simulink model "PMSG_Grid"  (R2023a)
settings: Solver=VariableStepAuto  StartTime=0.0  StopTime=4  FixedStep=1e-6  RelTol=1e-3  AbsTol=1e-3
libraries: slpidlib x6, spsabctodq0Lib x3, spsSVPWMGenerator2LevelLib x2, spsdq0toAlphaBetaZeroLib x2, spsUniversalBridgeLib x2, spsPermanentMagnetSynchronousMachineLib x1, spsPower3phInstantaneousLib x1, spspowerguiLib x1, spsSeriesRLCBranchLib x1, spsThreePhaseVIMeasurementLib x1, spsThreePhaseSourceLib x1, spsVoltageMeasurementLib x1
settings Model: Creator=MY  LastModifiedBy=MY

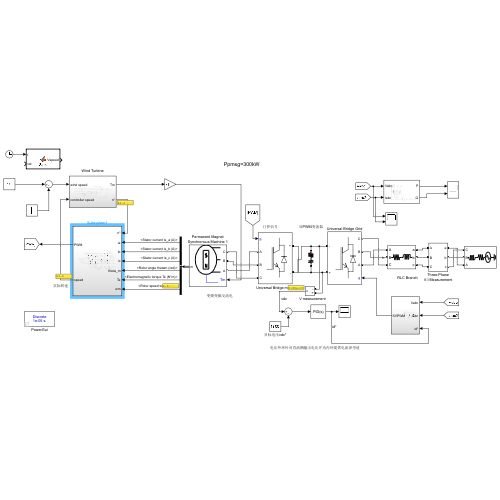
[thumbnail: Simulink's stored preview of the top-level diagram]
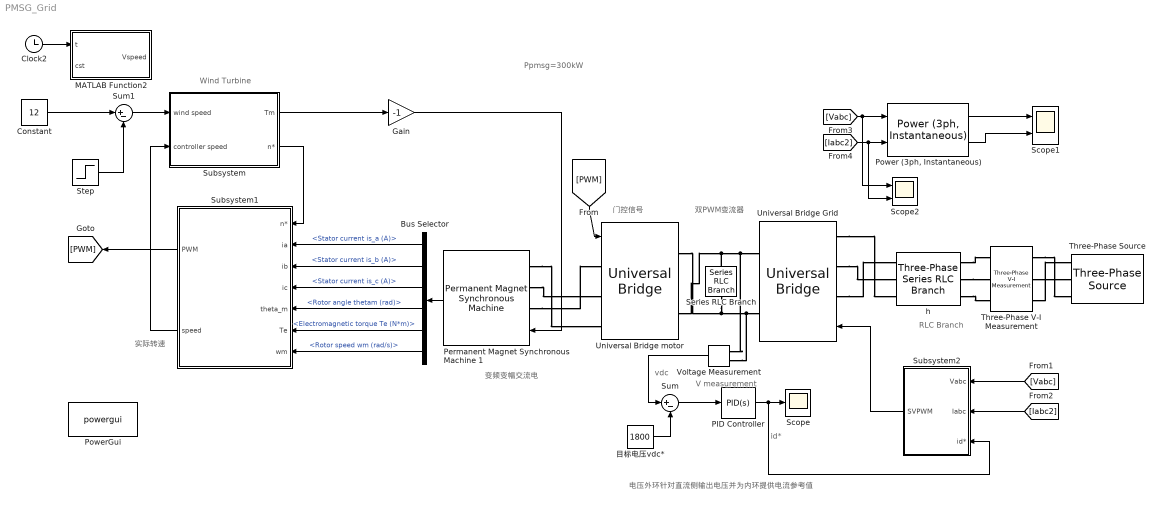
== system PMSG_Grid ==
  note: vdc
  note: 电压外环针对直流侧输出电压并为内环提供电流参考值
  note: 双PWM变流器
  note: 门控信号
  note: 变频变幅交流电
  note: 实际转速
  note: RLC Branch
  note: Ppmsg=300kW
  note: V measurement
  note: id*
  note: Wind Turbine
  Bus Selector : BusSelector  OutputSignals=Stator current is_a (A),Stator current is_b (A),Stator current is_c (A),Rotor angle thetam (rad),Electromagnetic torque Te (N*m),Rotor speed wm (rad/s)
  Clock2 : Clock
  Constant : Constant  Value=12
  Gain : Gain  Gain=-1
  MATLAB Function2 : MATLAB Function  InitFcn=""  StopFcn=""  TreatAsAtomicUnit=on
  PID Controller : slpidlib/PID Controller  Controller=PID  Form=Parallel  TimeDomain=Continuous-time  UseExternalTs=off  SampleTime=-1  IntegratorMethod=Forward Euler  FilterMethod=Forward Euler  ControllerParametersSource=internal  P=1  I=15  UseKiTs=off  D=0  N=100  UseFilter=on  TunerSelectOption=Transfer Function Based (PID Tuner App)  InitialConditionSource=internal  InitialConditionForIntegrator=0  InitialConditionForFilter=0  DifferentiatorICPrevScaledInput=0  ExternalReset=none  TrackingMode=off  Kt=1  LimitOutput=off  SatLimitsSource=internal  UpperSaturationLimit=inf  LowerSaturationLimit=-inf  LinearizeAsGain=on  AntiWindupMode=none  Kb=1  LimitIntegrator=off  UpperIntegratorSaturationLimit=inf  LowerIntegratorSaturationLimit=-inf  POutMin=[]  POutMax=[]  IOutMin=[]  IOutMax=[]  DOutMin=[]  DOutMax=[]  NOutMin=[]  NOutMax=[]  SumOutMin=[]  SumOutMax=[]  SaturationOutMin=[]  SaturationOutMax=[]  PParamMin=[]  PParamMax=[]  IParamMin=[]  IParamMax=[]  DParamMin=[]  DParamMax=[]  NParamMin=[]  NParamMax=[]  KbParamMin=[]  KbParamMax=[]  KtParamMin=[]  KtParamMax=[]  KbOutMin=[]  KbOutMax=[]  KtOutMin=[]  KtOutMax=[]  IntegratorOutMin=[]  IntegratorOutMax=[]  FilterOutMin=[]  FilterOutMax=[]  SumI1OutMin=[]  SumI1OutMax=[]  SumI2OutMin=[]  SumI2OutMax=[]  SumI3OutMin=[]  SumI3OutMax=[]  SumI4OutMin=[]  SumI4OutMax=[]  SumDOutMin=[]  SumDOutMax=[]  DifferentiatorOutMin=[]  DifferentiatorOutMax=[]  FilterDiffOutCoefMin=[]  FilterDiffOutCoefMax=[]  ReciprocalOutMin=[]  ReciprocalOutMax=[]  SumDenOutMin=[]  SumDenOutMax=[]  SumNumOutMin=[]  SumNumOutMax=[]  DivideOutMin=[]  DivideOutMax=[]  UdiffTsProdOutMin=[]  UdiffTsProdOutMax=[]  NTsProdOutMin=[]  NTsProdOutMax=[]  UintegralTsProdOutMin=[]  UintegralTsProdOutMax=[]  UngainTsProdOutMin=[]  UngainTsProdOutMax=[]  ClampingZeroOutDataTypeStr=Inherit: Inherit via back propagation  ClampingZeroOutMin=[]  ClampingZeroOutMax=[]  FilterDenConstantOutDataTypeStr=Inherit: Inherit via back propagation  FilterDenConstantOutMin=[]  FilterDenConstantOutMax=[]  PCopyOutDataTypeStr=Inherit: Inherit via back propagation  PCopyOutMin=[]  PCopyOutMax=[]  NCopyOutDataTypeStr=Inherit: Inherit via back propagation  NCopyOutMin=[]  NCopyOutMax=[]  IntegratorContinuousStateAttributes=''  IntegratorStateMustResolveToSignalObject=off  IntegratorRTWStateStorageClass=Auto  FilterContinuousStateAttributes=''  FilterStateMustResolveToSignalObject=off  FilterRTWStateStorageClass=Auto  ParallelPVariant=InternalParameters  IdealPVariant=Disabled  IVariant=InternalParameters  DVariant=InternalParameters  IntegratorVariant=Continuous  SatVariant=Disabled  AWVariant=Passthrough  PCopyVariant=Disabled  TRVariant=Disabled  FdbkBlocksVariant=Forward  IdealPFdbkVariant=Disabled  SatFdbkVariant=Disabled  DerivativeFilterVariant=ContFilter  NVariant=InternalParameters  NCopyVariant=Disabled  FilterICVariant=InternalICsFilter  IntegratorICVariant=InternalICs  ExternalResetVariant=Disabled  TRSumVariant=Passthrough  SumFdbkVariant=Disabled  SumVariant=Sum_PID  TsampFilterVariant=InternalTs  TsampNgainVariant=Passthrough  TsampIntegralVariant=Disabled_SignalSpec  ExternalSaturationOutDataTypeStr=Inherit: Same as second input
  Permanent Magnet Synchronous Machine 1 : spsPermanentMagnetSynchronousMachineLib/Permanent Magnet Synchronous Machine  NbPhases=3  FluxDistribution=Sinusoidal  RotorType=Round  MechanicalLoad=Torque Tm  PresetModel=No  ShowDetailedParameters=on  MeasurementBus=off  Resistance=0.025  Inductance=8.5e-3  dqInductances=[8.5e-3,8.5e-3]  La=0.0036  MachineConstant=Flux linkage established by magnets (V.s)  Flux=3.88889  VoltageCst=8464.3995  TorqueCst=70  Flat=120  Mechanical=[60 0.078 12 0]  PolePairs=4  InitialConditions=[0,0, 0,0]  InitialConditions5ph=[0 0 0 0 0 0]  RefAngle=90 degrees behind phase A axis (modified Park)  IterativeDiscreteModel=Trapezoidal non iterative  TsBlock=-1  TsPowergui=0
  "Power (3ph, Instantaneous)" : spsPower3phInstantaneousLib/Power (3ph, Instantaneous)
  PowerGui : spspowerguiLib/powergui  Priority=1  SimulationMode=Discrete  SampleTime=1e-5  frequency=60  Iterations=50  frequencyindice=60  Pbase=100e6  ErrMax=1e-4  UnitsV=kV  UnitsW=MW  buscounter=0  FunctionMessages=off  echomessages=off  EnableUseOfTLC=off  CurrentSourceSwitches=off  DisableSnubberDevices=off  DisableRonSwitches=off  DisableVfSwitches=off  DisplayEquations=off  AutomaticDiscreteSolvers=off  SolverType=Tustin/Backward Euler (TBE)  Interpol=off  ExternalGateDelay=off  methode=off  Ts=100  x0status=blocks  SPID=on  SwTol=0  HookPort=off  NonlinearTolerance=1e-4  nMaxIteration=100  ContinueOnMaxIteration=off  RestoreLinks=warning  ResistiveCurrentMeasurement=off  Frange=[0:2:500]  Ylog=off  Xlog=on  ShowGrid=off  save=off  variable=ZData  structure=0  ZoomFFT=off  StartTime=0.0  cycles=1  DisplayStyle=1  fundamental=60  FreqAxis=off  MaxFrequency=1000  frequencyindicesteady=1  RmsSteady=1  display=off
  Scope : Scope
  Scope1 : Scope  NumInputPorts=2
  Scope2 : Scope  NumInputPorts=2
  Series RLC Branch : spsSeriesRLCBranchLib/Series RLC Branch  LConnTagsString=__new0  RConnTagsString=__new0  BranchType=RC  Resistance=1  Inductance=1e-3  SetiL0=off  InitialCurrent=0  Capacitance=1e-3  Setx0=off  InitialVoltage=0  Measurements=None
  Step : Step  Time=1.5  After=4  SampleTime=0
  Subsystem : Subsystem
  Subsystem1 : Subsystem
  Subsystem2 : Subsystem
  Sum : Sum  Inputs=|+-
  Sum1 : Sum  Inputs=|+-
  "Three-Phase V-I Measurement " : spsThreePhaseVIMeasurementLib/Three-Phase V-I Measurement  VoltageMeasurement=phase-to-phase  SetLabelV=on  LabelV=Vabc  Vpu=off  VpuLL=off  CurrentMeasurement=yes  SetLabelI=on  LabelI=Iabc2  Ipu=off  Pbase=100e6  Vbase=500e3  OutputType=Complex  PhasorSimulation=off  PSBequivalent=0
  Three-Phase Source : spsThreePhaseSourceLib/Three-Phase Source  InternalConnection=Yg  VoltagePhases=off  Voltage=690  PhaseAngle=0  Voltage_phases=[25e3 25e3 25e3]/sqrt(3)  PhaseAngles_phases=[0 -120 +120]  Frequency=60  NonIdealSource=on  SpecifyImpedance=off  Resistance=0.8929  Inductance=16.58e-3  ShortCircuitLevel=100e6  BaseVoltage=25e3  XRratio=7  BusType=swing  Pref=10e3  Qref=0  Prefabc=[10e3, 10e3, 10e3]  Qrefabc=[0, 0, 0]  Qmin=-inf  Qmax=inf
  Universal Bridge Grid : spsUniversalBridgeLib/Universal Bridge  Arms=3  SnubberResistance=1e5  SnubberCapacitance=inf  Device=IGBT / Diodes  Ron=1e-3  Lon=0  ForwardVoltages="[  0  0  ]"  ForwardVoltage=0  GTOparameters=[ 10e-6 , 20e-6 ]  IGBTparameters=[ 1e-6 , 2e-6 ]  Measurements=All voltages and currents  Measurements_2=None  converterType=Rectifier
  Universal Bridge motor : spsUniversalBridgeLib/Universal Bridge  Arms=3  SnubberResistance=1e5  SnubberCapacitance=inf  Device=IGBT / Diodes  Ron=1e-3  Lon=0  ForwardVoltages="[  0  0  ]"  ForwardVoltage=0  GTOparameters=[ 10e-6 , 20e-6 ]  IGBTparameters=[ 1e-6 , 2e-6 ]  Measurements=All voltages and currents  Measurements_2=None  converterType=Rectifier
  Voltage Measurement : spsVoltageMeasurementLib/Voltage Measurement  PhasorSimulation=off  OutputType=Complex  PSBequivalent=0
  "h " : spsThreePhaseSeriesRLCBranchLib/Three-Phase Series RLC Branch  LConnTagsString=A|B|C  RConnTagsString=A|B|C  BranchType=RL  Resistance=1  Inductance=1e-3  Capacitance=1e-6  Measurements=None
  目标电压vdc* : Constant  Value=1800
  wires:
  Permanent Magnet Synchronous Machine 1/1 -> Bus Selector/1
  Bus Selector/1 -> Subsystem1/2(ia)  "<Stator current is_a (A)>"
  Bus Selector/2 -> Subsystem1/3(ib)  "<Stator current is_b (A)>"
  Bus Selector/3 -> Subsystem1/4(ic)  "<Stator current is_c (A)>"
  Bus Selector/4 -> Subsystem1/5(theta_m)  "<Rotor angle thetam (rad)>"
  Bus Selector/5 -> Subsystem1/6(Te)  "<Electromagnetic torque Te (N*m)>"
  Bus Selector/6 -> Subsystem1/7(wm)  "<Rotor speed wm (rad/s)>"
  [PWM] -> Universal Bridge motor/1
  Sum/1 -> PID Controller/1
  目标电压vdc*/1 -> Sum/2
  Voltage Measurement/1 -> Sum/1
  PID Controller/1 -> Subsystem2/3(id*), Scope/1
  Subsystem2/1(SVPWM) -> Universal Bridge Grid/1
  [Vabc] -> Subsystem2/1(Vabc)
  [Iabc2] -> Subsystem2/2(Iabc)
  Subsystem1/1(PWM) -> [PWM]
  [Vabc] -> Scope2/1, "Power (3ph, Instantaneous)"/1
  [Iabc2] -> Scope2/2, "Power (3ph, Instantaneous)"/2
  "Power (3ph, Instantaneous)"/1 -> Scope1/1
  "Power (3ph, Instantaneous)"/2 -> Scope1/2
  Step/1 -> Sum1/2
  Gain/1 -> Permanent Magnet Synchronous Machine 1/1
  Subsystem/1(Tm) -> Gain/1
  Subsystem/2(n*) -> Subsystem1/1(n*)
  Subsystem1/2(speed) -> Subsystem/2(controller speed)
  Clock2/1 -> MATLAB Function2/1(t)
  Constant/1 -> Sum1/1
  Sum1/1 -> Subsystem/1(wind speed)
  connections:
  Universal Bridge Grid/LConn1 -- "h "/LConn1
  Universal Bridge Grid/LConn2 -- "h "/LConn2
  "h "/RConn1 -- "Three-Phase V-I Measurement "/LConn1
  "h "/RConn2 -- "Three-Phase V-I Measurement "/LConn2
  "h "/RConn3 -- "Three-Phase V-I Measurement "/LConn3
  "Three-Phase V-I Measurement "/RConn1 -- Three-Phase Source/RConn1
  "Three-Phase V-I Measurement "/RConn2 -- Three-Phase Source/RConn2
  "Three-Phase V-I Measurement "/RConn3 -- Three-Phase Source/RConn3
  Permanent Magnet Synchronous Machine 1/LConn1 -- Universal Bridge motor/LConn1
  Permanent Magnet Synchronous Machine 1/LConn2 -- Universal Bridge motor/LConn2
  Permanent Magnet Synchronous Machine 1/LConn3 -- Universal Bridge motor/LConn3
  Universal Bridge Grid/LConn3 -- "h "/LConn3
  Universal Bridge motor/RConn1 -- Series RLC Branch/RConn1 -- Voltage Measurement/LConn1 -- Universal Bridge Grid/RConn1
  Universal Bridge motor/RConn2 -- Series RLC Branch/LConn1 -- Voltage Measurement/LConn2 -- Universal Bridge Grid/RConn2

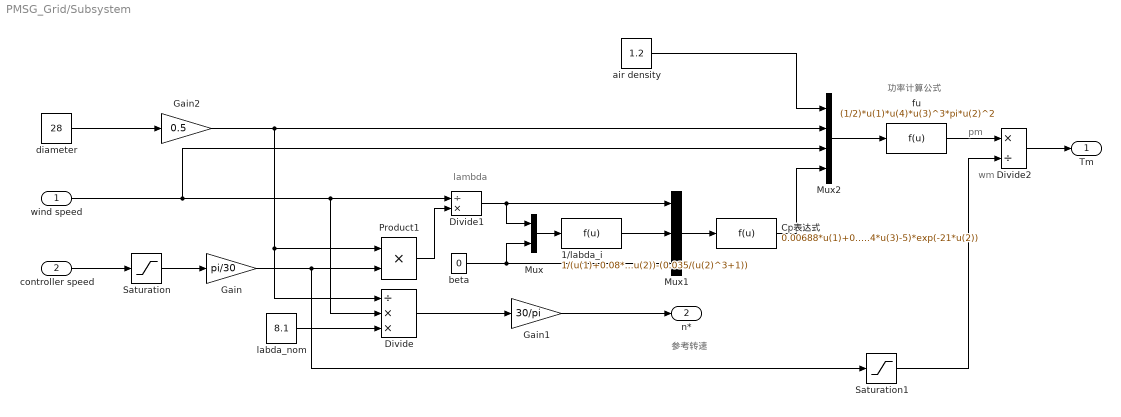
== system PMSG_Grid/Subsystem ==
  note: 参考转速
  note: 功率计算公式
  note: pm
  note: wm
  note: lambda
  wind speed : Inport
  controller speed : Inport  Port=2
  1/labda_i : Fcn  Expr=1/(u(1)+0.08*u(2))-(0.035/(u(2)^3+1))
  Cp表达式 : Fcn  Expr=0.00688*u(1)+0.5176*(116*u(2)-0.4*u(3)-5)*exp(-21*u(2))
  Divide : Product  Inputs=/**
  Divide1 : Product  Inputs=/*
  Divide2 : Product  Inputs=*/
  Gain : Gain  Gain=pi/30
  Gain1 : Gain  Gain=30/pi
  Gain2 : Gain  Gain=0.5
  Mux : Mux  Inputs=2
  Mux1 : Mux  Inputs=3
  Mux2 : Mux
  Product1 : Product
  Saturation : Saturate  UpperLimit=1e5  LowerLimit=1e-5
  Saturation1 : Saturate  UpperLimit=1e5  LowerLimit=1e-5
  air density : Constant  Value=1.2
  beta : Constant  Value=0
  diameter : Constant  Value=28
  fu : Fcn  Expr=(1/2)*u(1)*u(4)*u(3)^3*pi*u(2)^2
  labda_nom : Constant  Value=8.1
  Tm : Outport
  n* : Outport  Port=2
  wires:
  Gain1/1 -> n*/1
  Gain/1 -> Saturation1/1, Product1/2
  Divide/1 -> Gain1/1
  beta/1 -> Mux/2, Mux1/3
  wind speed/1 -> Divide/2, Divide1/1, Mux2/3
  diameter/1 -> Gain2/1
  Divide1/1 -> Mux/1, Mux1/1
  Gain2/1 -> Divide/1, Product1/1, Mux2/2
  1/labda_i/1 -> Mux1/2
  Saturation/1 -> Gain/1
  labda_nom/1 -> Divide/3
  Product1/1 -> Divide1/2
  Mux/1 -> 1/labda_i/1
  controller speed/1 -> Saturation/1
  Mux1/1 -> Cp表达式/1
  Cp表达式/1 -> Mux2/4
  air density/1 -> Mux2/1
  Mux2/1 -> fu/1
  fu/1 -> Divide2/1
  Saturation1/1 -> Divide2/2
  Divide2/1 -> Tm/1

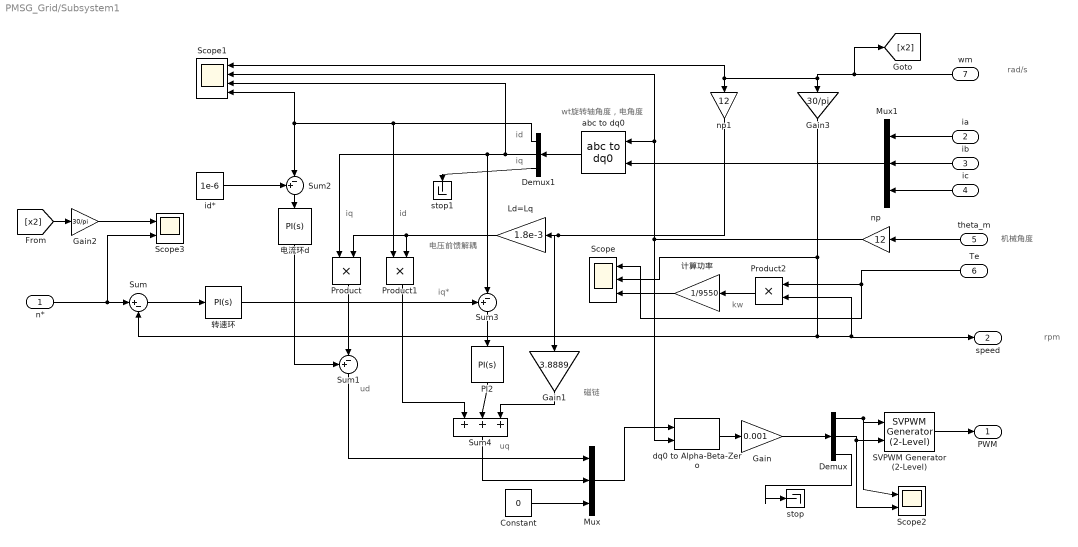
== system PMSG_Grid/Subsystem1 ==
  note: kw
  note: rpm
  note: rad/s
  note: 电压前馈解耦
  note: 磁链
  note: ud
  note: uq
  note: iq*
  note: 机械角度
  note: wt旋转轴角度，电角度
  note: id
  note: iq
  note: iq
  note: id
  n* : Inport
  ia : Inport  Port=2
  ib : Inport  Port=3
  ic : Inport  Port=4
  theta_m : Inport  Port=5
  Te : Inport  Port=6
  wm : Inport  Port=7
  Constant : Constant  Value=0
  Demux : Demux  Outputs=3
  Demux1 : Demux  Outputs=3
  Gain : Gain  Gain=0.001
  Gain1 : Gain  Gain=3.8889
  Gain2 : Gain  Gain=30/pi
  Gain3 : Gain  Gain=30/pi
  "Ld=Lq " : Gain  Gain=1.8e-3
  Mux : Mux  Inputs=3
  Mux1 : Mux  Inputs=3
  PI2 : slpidlib/PID Controller  Controller=PI  Form=Parallel  TimeDomain=Continuous-time  UseExternalTs=off  SampleTime=-1  IntegratorMethod=Forward Euler  FilterMethod=Forward Euler  ControllerParametersSource=internal  P=1  I=12  UseKiTs=off  D=0  N=100  UseFilter=on  TunerSelectOption=Transfer Function Based (PID Tuner App)  InitialConditionSource=internal  InitialConditionForIntegrator=0  InitialConditionForFilter=0  DifferentiatorICPrevScaledInput=0  ExternalReset=none  TrackingMode=off  Kt=1  LimitOutput=off  SatLimitsSource=internal  UpperSaturationLimit=inf  LowerSaturationLimit=-inf  LinearizeAsGain=on  AntiWindupMode=none  Kb=1  LimitIntegrator=off  UpperIntegratorSaturationLimit=inf  LowerIntegratorSaturationLimit=-inf  POutMin=[]  POutMax=[]  IOutMin=[]  IOutMax=[]  DOutMin=[]  DOutMax=[]  NOutMin=[]  NOutMax=[]  SumOutMin=[]  SumOutMax=[]  SaturationOutMin=[]  SaturationOutMax=[]  PParamMin=[]  PParamMax=[]  IParamMin=[]  IParamMax=[]  DParamMin=[]  DParamMax=[]  NParamMin=[]  NParamMax=[]  KbParamMin=[]  KbParamMax=[]  KtParamMin=[]  KtParamMax=[]  KbOutMin=[]  KbOutMax=[]  KtOutMin=[]  KtOutMax=[]  IntegratorOutMin=[]  IntegratorOutMax=[]  FilterOutMin=[]  FilterOutMax=[]  SumI1OutMin=[]  SumI1OutMax=[]  SumI2OutMin=[]  SumI2OutMax=[]  SumI3OutMin=[]  SumI3OutMax=[]  SumI4OutMin=[]  SumI4OutMax=[]  SumDOutMin=[]  SumDOutMax=[]  DifferentiatorOutMin=[]  DifferentiatorOutMax=[]  FilterDiffOutCoefMin=[]  FilterDiffOutCoefMax=[]  ReciprocalOutMin=[]  ReciprocalOutMax=[]  SumDenOutMin=[]  SumDenOutMax=[]  SumNumOutMin=[]  SumNumOutMax=[]  DivideOutMin=[]  DivideOutMax=[]  UdiffTsProdOutMin=[]  UdiffTsProdOutMax=[]  NTsProdOutMin=[]  NTsProdOutMax=[]  UintegralTsProdOutMin=[]  UintegralTsProdOutMax=[]  UngainTsProdOutMin=[]  UngainTsProdOutMax=[]  ClampingZeroOutDataTypeStr=Inherit: Inherit via back propagation  ClampingZeroOutMin=[]  ClampingZeroOutMax=[]  FilterDenConstantOutDataTypeStr=Inherit: Inherit via back propagation  FilterDenConstantOutMin=[]  FilterDenConstantOutMax=[]  PCopyOutDataTypeStr=Inherit: Inherit via back propagation  PCopyOutMin=[]  PCopyOutMax=[]  NCopyOutDataTypeStr=Inherit: Inherit via back propagation  NCopyOutMin=[]  NCopyOutMax=[]  IntegratorContinuousStateAttributes=''  IntegratorStateMustResolveToSignalObject=off  IntegratorRTWStateStorageClass=Auto  FilterContinuousStateAttributes=''  FilterStateMustResolveToSignalObject=off  FilterRTWStateStorageClass=Auto  ParallelPVariant=InternalParameters  IdealPVariant=Disabled  IVariant=InternalParameters  DVariant=Disabled  IntegratorVariant=Continuous  SatVariant=Disabled  AWVariant=Passthrough  PCopyVariant=Disabled  TRVariant=Disabled  FdbkBlocksVariant=Forward  IdealPFdbkVariant=Disabled  SatFdbkVariant=Disabled  DerivativeFilterVariant=Disabled  NVariant=Disabled  NCopyVariant=Disabled_SignalSpec  FilterICVariant=Disabled  IntegratorICVariant=InternalICs  ExternalResetVariant=Disabled  TRSumVariant=Passthrough  SumFdbkVariant=Disabled  SumVariant=Sum_PI  TsampFilterVariant=InternalTs  TsampNgainVariant=Passthrough  TsampIntegralVariant=Disabled_SignalSpec  ExternalSaturationOutDataTypeStr=Inherit: Same as second input
  Product : Product
  Product1 : Product
  Product2 : Product
  SVPWM Generator (2-Level) : spsSVPWMGenerator2LevelLib/SVPWM Generator (2-Level)  InputType=alpha-beta components  SwitchingPattern=Pattern #1  Fc=3000  ParUref=[0.8 -30 50]  Ts=0
  Scope : Scope  NumInputPorts=3
  Scope1 : Scope  NumInputPorts=4
  Scope2 : Scope  NumInputPorts=2
  Scope3 : Scope  NumInputPorts=2
  Sum : Sum  Inputs=|+-
  Sum1 : Sum  Inputs=+-|
  Sum2 : Sum  Inputs=+-|
  Sum3 : Sum  Inputs=+-|
  Sum4 : Sum  Inputs=+|++
  abc to dq0 : spsabctodq0Lib/abc to dq0  Alignment=90 degrees behind phase A axis
  dq0 to Alpha-Beta-Zero : spsdq0toAlphaBetaZeroLib/dq0 to Alpha-Beta-Zero  Alignment=90 degrees behind phase A axis
  id* : Constant  Value=1e-6
  np : Gain  Gain=12
  np1 : Gain  Gain=12
  stop : Terminator
  stop1 : Terminator
  电流环d : slpidlib/PID Controller  Controller=PI  Form=Parallel  TimeDomain=Continuous-time  UseExternalTs=off  SampleTime=-1  IntegratorMethod=Forward Euler  FilterMethod=Forward Euler  ControllerParametersSource=internal  P=1  I=12  UseKiTs=on  D=0  N=100  UseFilter=on  TunerSelectOption=Frequency Response Based  ZeroCross=off  InitialConditionSource=internal  InitialConditionForIntegrator=0  InitialConditionForFilter=0  DifferentiatorICPrevScaledInput=0  ExternalReset=none  TrackingMode=off  Kt=1  LimitOutput=off  SatLimitsSource=internal  UpperSaturationLimit=inf  LowerSaturationLimit=-inf  LinearizeAsGain=on  AntiWindupMode=none  Kb=1  LimitIntegrator=off  UpperIntegratorSaturationLimit=inf  LowerIntegratorSaturationLimit=-inf  POutMin=[]  POutMax=[]  IOutMin=[]  IOutMax=[]  DOutMin=[]  DOutMax=[]  NOutMin=[]  NOutMax=[]  SumOutMin=[]  SumOutMax=[]  SaturationOutMin=[]  SaturationOutMax=[]  PParamMin=[]  PParamMax=[]  IParamMin=[]  IParamMax=[]  DParamMin=[]  DParamMax=[]  NParamMin=[]  NParamMax=[]  KbParamMin=[]  KbParamMax=[]  KtParamMin=[]  KtParamMax=[]  KbOutMin=[]  KbOutMax=[]  KtOutMin=[]  KtOutMax=[]  IntegratorOutMin=[]  IntegratorOutMax=[]  FilterOutMin=[]  FilterOutMax=[]  SumI1OutMin=[]  SumI1OutMax=[]  SumI2OutMin=[]  SumI2OutMax=[]  SumI3OutMin=[]  SumI3OutMax=[]  SumI4OutMin=[]  SumI4OutMax=[]  SumDOutMin=[]  SumDOutMax=[]  DifferentiatorOutMin=[]  DifferentiatorOutMax=[]  FilterDiffOutCoefMin=[]  FilterDiffOutCoefMax=[]  ReciprocalOutMin=[]  ReciprocalOutMax=[]  SumDenOutMin=[]  SumDenOutMax=[]  SumNumOutMin=[]  SumNumOutMax=[]  DivideOutMin=[]  DivideOutMax=[]  UdiffTsProdOutMin=[]  UdiffTsProdOutMax=[]  NTsProdOutMin=[]  NTsProdOutMax=[]  UintegralTsProdOutMin=[]  UintegralTsProdOutMax=[]  UngainTsProdOutMin=[]  UngainTsProdOutMax=[]  ClampingZeroOutDataTypeStr=Inherit: Inherit via back propagation  ClampingZeroOutMin=[]  ClampingZeroOutMax=[]  FilterDenConstantOutDataTypeStr=Inherit: Inherit via back propagation  FilterDenConstantOutMin=[]  FilterDenConstantOutMax=[]  PCopyOutDataTypeStr=Inherit: Inherit via back propagation  PCopyOutMin=[]  PCopyOutMax=[]  NCopyOutDataTypeStr=Inherit: Inherit via back propagation  NCopyOutMin=[]  NCopyOutMax=[]  IntegratorContinuousStateAttributes=''  IntegratorStateMustResolveToSignalObject=off  IntegratorRTWStateStorageClass=Auto  FilterContinuousStateAttributes=''  FilterStateMustResolveToSignalObject=off  FilterRTWStateStorageClass=Auto  ParallelPVariant=InternalParameters  IdealPVariant=Disabled  IVariant=InternalParameters  DVariant=Disabled  IntegratorVariant=Continuous  SatVariant=Disabled  AWVariant=Passthrough  PCopyVariant=Disabled  TRVariant=Disabled  FdbkBlocksVariant=Forward  IdealPFdbkVariant=Disabled  SatFdbkVariant=Disabled  DerivativeFilterVariant=Disabled  NVariant=Disabled  NCopyVariant=Disabled_SignalSpec  FilterICVariant=Disabled  IntegratorICVariant=InternalICs  ExternalResetVariant=Disabled  TRSumVariant=Passthrough  SumFdbkVariant=Disabled  SumVariant=Sum_PI  TsampFilterVariant=InternalTs  TsampNgainVariant=Passthrough  TsampIntegralVariant=Disabled_SignalSpec  ExternalSaturationOutDataTypeStr=Inherit: Same as second input
  计算功率 : Gain  Gain=1/9550
  转速环 : slpidlib/PID Controller  Controller=PI  Form=Parallel  TimeDomain=Continuous-time  UseExternalTs=off  SampleTime=-1  IntegratorMethod=Forward Euler  FilterMethod=Forward Euler  ControllerParametersSource=internal  P=10  I=220  UseKiTs=off  D=0  N=100  UseFilter=on  TunerSelectOption=Transfer Function Based (PID Tuner App)  InitialConditionSource=internal  InitialConditionForIntegrator=0  InitialConditionForFilter=0  DifferentiatorICPrevScaledInput=0  ExternalReset=none  TrackingMode=off  Kt=1  LimitOutput=off  SatLimitsSource=internal  UpperSaturationLimit=inf  LowerSaturationLimit=-inf  LinearizeAsGain=on  AntiWindupMode=none  Kb=1  LimitIntegrator=off  UpperIntegratorSaturationLimit=inf  LowerIntegratorSaturationLimit=-inf  POutMin=[]  POutMax=[]  IOutMin=[]  IOutMax=[]  DOutMin=[]  DOutMax=[]  NOutMin=[]  NOutMax=[]  SumOutMin=[]  SumOutMax=[]  SaturationOutMin=[]  SaturationOutMax=[]  PParamMin=[]  PParamMax=[]  IParamMin=[]  IParamMax=[]  DParamMin=[]  DParamMax=[]  NParamMin=[]  NParamMax=[]  KbParamMin=[]  KbParamMax=[]  KtParamMin=[]  KtParamMax=[]  KbOutMin=[]  KbOutMax=[]  KtOutMin=[]  KtOutMax=[]  IntegratorOutMin=[]  IntegratorOutMax=[]  FilterOutMin=[]  FilterOutMax=[]  SumI1OutMin=[]  SumI1OutMax=[]  SumI2OutMin=[]  SumI2OutMax=[]  SumI3OutMin=[]  SumI3OutMax=[]  SumI4OutMin=[]  SumI4OutMax=[]  SumDOutMin=[]  SumDOutMax=[]  DifferentiatorOutMin=[]  DifferentiatorOutMax=[]  FilterDiffOutCoefMin=[]  FilterDiffOutCoefMax=[]  ReciprocalOutMin=[]  ReciprocalOutMax=[]  SumDenOutMin=[]  SumDenOutMax=[]  SumNumOutMin=[]  SumNumOutMax=[]  DivideOutMin=[]  DivideOutMax=[]  UdiffTsProdOutMin=[]  UdiffTsProdOutMax=[]  NTsProdOutMin=[]  NTsProdOutMax=[]  UintegralTsProdOutMin=[]  UintegralTsProdOutMax=[]  UngainTsProdOutMin=[]  UngainTsProdOutMax=[]  ClampingZeroOutDataTypeStr=Inherit: Inherit via back propagation  ClampingZeroOutMin=[]  ClampingZeroOutMax=[]  FilterDenConstantOutDataTypeStr=Inherit: Inherit via back propagation  FilterDenConstantOutMin=[]  FilterDenConstantOutMax=[]  PCopyOutDataTypeStr=Inherit: Inherit via back propagation  PCopyOutMin=[]  PCopyOutMax=[]  NCopyOutDataTypeStr=Inherit: Inherit via back propagation  NCopyOutMin=[]  NCopyOutMax=[]  IntegratorContinuousStateAttributes=''  IntegratorStateMustResolveToSignalObject=off  IntegratorRTWStateStorageClass=Auto  FilterContinuousStateAttributes=''  FilterStateMustResolveToSignalObject=off  FilterRTWStateStorageClass=Auto  ParallelPVariant=InternalParameters  IdealPVariant=Disabled  IVariant=InternalParameters  DVariant=Disabled  IntegratorVariant=Continuous  SatVariant=Disabled  AWVariant=Passthrough  PCopyVariant=Disabled  TRVariant=Disabled  FdbkBlocksVariant=Forward  IdealPFdbkVariant=Disabled  SatFdbkVariant=Disabled  DerivativeFilterVariant=Disabled  NVariant=Disabled  NCopyVariant=Disabled_SignalSpec  FilterICVariant=Disabled  IntegratorICVariant=InternalICs  ExternalResetVariant=Disabled  TRSumVariant=Passthrough  SumFdbkVariant=Disabled  SumVariant=Sum_PI  TsampFilterVariant=InternalTs  TsampNgainVariant=Passthrough  TsampIntegralVariant=Disabled_SignalSpec  ExternalSaturationOutDataTypeStr=Inherit: Same as second input
  PWM : Outport
  speed : Outport  Port=2
  wires:
  n*/1 -> Scope3/2, Sum/1
  Sum/1 -> 转速环/1
  Sum3/1 -> PI2/1
  PI2/1 -> Sum4/2
  Sum1/1 -> Mux/1
  Sum4/1 -> Mux/2
  Constant/1 -> Mux/3
  Product/1 -> Sum1/2
  Product1/1 -> Sum4/1
  Mux/1 -> dq0 to Alpha-Beta-Zero/1
  dq0 to Alpha-Beta-Zero/1 -> Gain/1
  Gain/1 -> Demux/1
  Demux/2 -> Scope2/2, SVPWM Generator (2-Level)/2
  Demux/1 -> Scope2/1, SVPWM Generator (2-Level)/1
  SVPWM Generator (2-Level)/1 -> PWM/1
  Gain1/1 -> Sum4/3
  "Ld=Lq "/1 -> Product1/2, Product/2
  Demux1/3 -> stop1/1
  Demux1/2 -> Scope1/3, Product/1, Sum3/2
  abc to dq0/1 -> Demux1/1
  ia/1 -> Mux1/1
  ib/1 -> Mux1/2
  ic/1 -> Mux1/3
  Mux1/1 -> abc to dq0/1
  theta_m/1 -> np/1
  np/1 -> dq0 to Alpha-Beta-Zero/2, Scope1/2, abc to dq0/2
  wm/1 -> [x2], Scope1/1, np1/1, Gain3/1
  Gain3/1 -> Scope/2, Product2/2, speed/1, Sum/2
  Te/1 -> Scope/1, Product2/1
  Product2/1 -> 计算功率/1
  计算功率/1 -> Scope/3
  np1/1 -> "Ld=Lq "/1, Gain1/1
  Demux/3 -> stop/1
  Demux1/1 -> Product1/1, Scope1/4, Sum2/2
  id*/1 -> Sum2/1
  Sum2/1 -> 电流环d/1
  电流环d/1 -> Sum1/1
  转速环/1 -> Sum3/1
  [x2] -> Gain2/1
  Gain2/1 -> Scope3/1

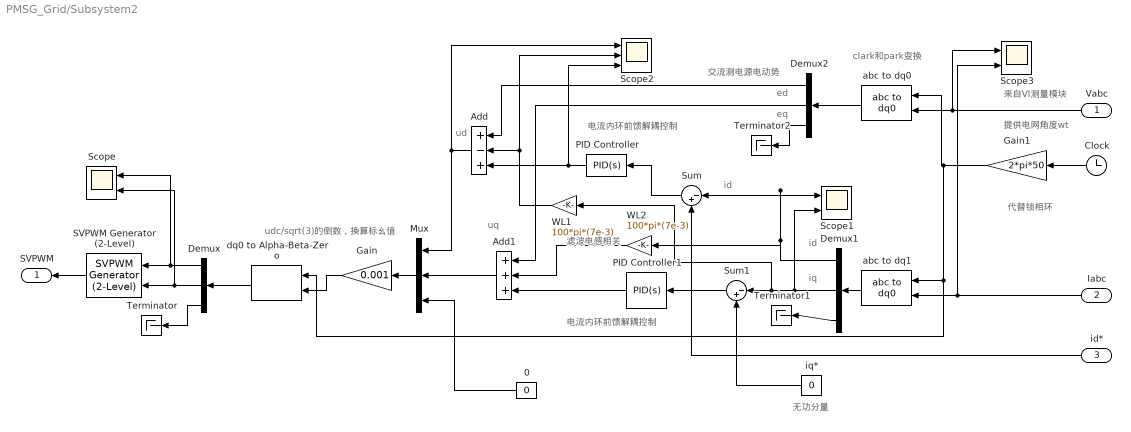
== system PMSG_Grid/Subsystem2 ==
  note: udc/sqrt(3)的倒数，换算标幺值
  note: 无功分量
  note: 电流内环前馈解耦控制
  note: 交流测电源电动势
  note: 提供电网角度wt
  note: clark和park变换
  note: 滤波电感相关
  note: 来自VI测量模块
  note: ed
  note: eq
  note: iq
  note: id
  note: uq
  note: 代替锁相环
  note: ud
  note: id
  note: 电流内环前馈解耦控制
  Vabc : Inport
  Iabc : Inport  Port=2
  id* : Inport  Port=3
  0 : Constant  Value=0
  Add : Sum  Inputs=+-+
  Add1 : Sum  Inputs=+++
  Clock : Clock
  Demux : Demux  Outputs=3
  Demux1 : Demux  Outputs=3
  Demux2 : Demux  Outputs=3
  Gain : Gain  Gain=0.001
  Gain1 : Gain  Gain=2*pi*50
  Mux : Mux  Inputs=3
  PID Controller : slpidlib/PID Controller  Controller=PID  Form=Parallel  TimeDomain=Continuous-time  UseExternalTs=off  SampleTime=-1  IntegratorMethod=Forward Euler  FilterMethod=Forward Euler  ControllerParametersSource=internal  P=1  I=15  UseKiTs=off  D=0  N=100  UseFilter=on  TunerSelectOption=Transfer Function Based (PID Tuner App)  InitialConditionSource=internal  InitialConditionForIntegrator=0  InitialConditionForFilter=0  DifferentiatorICPrevScaledInput=0  ExternalReset=none  TrackingMode=off  Kt=1  LimitOutput=off  SatLimitsSource=internal  UpperSaturationLimit=inf  LowerSaturationLimit=-inf  LinearizeAsGain=on  AntiWindupMode=none  Kb=1  LimitIntegrator=off  UpperIntegratorSaturationLimit=inf  LowerIntegratorSaturationLimit=-inf  POutMin=[]  POutMax=[]  IOutMin=[]  IOutMax=[]  DOutMin=[]  DOutMax=[]  NOutMin=[]  NOutMax=[]  SumOutMin=[]  SumOutMax=[]  SaturationOutMin=[]  SaturationOutMax=[]  PParamMin=[]  PParamMax=[]  IParamMin=[]  IParamMax=[]  DParamMin=[]  DParamMax=[]  NParamMin=[]  NParamMax=[]  KbParamMin=[]  KbParamMax=[]  KtParamMin=[]  KtParamMax=[]  KbOutMin=[]  KbOutMax=[]  KtOutMin=[]  KtOutMax=[]  IntegratorOutMin=[]  IntegratorOutMax=[]  FilterOutMin=[]  FilterOutMax=[]  SumI1OutMin=[]  SumI1OutMax=[]  SumI2OutMin=[]  SumI2OutMax=[]  SumI3OutMin=[]  SumI3OutMax=[]  SumI4OutMin=[]  SumI4OutMax=[]  SumDOutMin=[]  SumDOutMax=[]  DifferentiatorOutMin=[]  DifferentiatorOutMax=[]  FilterDiffOutCoefMin=[]  FilterDiffOutCoefMax=[]  ReciprocalOutMin=[]  ReciprocalOutMax=[]  SumDenOutMin=[]  SumDenOutMax=[]  SumNumOutMin=[]  SumNumOutMax=[]  DivideOutMin=[]  DivideOutMax=[]  UdiffTsProdOutMin=[]  UdiffTsProdOutMax=[]  NTsProdOutMin=[]  NTsProdOutMax=[]  UintegralTsProdOutMin=[]  UintegralTsProdOutMax=[]  UngainTsProdOutMin=[]  UngainTsProdOutMax=[]  ClampingZeroOutDataTypeStr=Inherit: Inherit via back propagation  ClampingZeroOutMin=[]  ClampingZeroOutMax=[]  FilterDenConstantOutDataTypeStr=Inherit: Inherit via back propagation  FilterDenConstantOutMin=[]  FilterDenConstantOutMax=[]  PCopyOutDataTypeStr=Inherit: Inherit via back propagation  PCopyOutMin=[]  PCopyOutMax=[]  NCopyOutDataTypeStr=Inherit: Inherit via back propagation  NCopyOutMin=[]  NCopyOutMax=[]  IntegratorContinuousStateAttributes=''  IntegratorStateMustResolveToSignalObject=off  IntegratorRTWStateStorageClass=Auto  FilterContinuousStateAttributes=''  FilterStateMustResolveToSignalObject=off  FilterRTWStateStorageClass=Auto  ParallelPVariant=InternalParameters  IdealPVariant=Disabled  IVariant=InternalParameters  DVariant=InternalParameters  IntegratorVariant=Continuous  SatVariant=Disabled  AWVariant=Passthrough  PCopyVariant=Disabled  TRVariant=Disabled  FdbkBlocksVariant=Forward  IdealPFdbkVariant=Disabled  SatFdbkVariant=Disabled  DerivativeFilterVariant=ContFilter  NVariant=InternalParameters  NCopyVariant=Disabled  FilterICVariant=InternalICsFilter  IntegratorICVariant=InternalICs  ExternalResetVariant=Disabled  TRSumVariant=Passthrough  SumFdbkVariant=Disabled  SumVariant=Sum_PID  TsampFilterVariant=InternalTs  TsampNgainVariant=Passthrough  TsampIntegralVariant=Disabled_SignalSpec  ExternalSaturationOutDataTypeStr=Inherit: Same as second input
  PID Controller1 : slpidlib/PID Controller  Controller=PID  Form=Parallel  TimeDomain=Continuous-time  UseExternalTs=off  SampleTime=-1  IntegratorMethod=Forward Euler  FilterMethod=Forward Euler  ControllerParametersSource=internal  P=1  I=15  UseKiTs=off  D=0  N=100  UseFilter=on  TunerSelectOption=Transfer Function Based (PID Tuner App)  InitialConditionSource=internal  InitialConditionForIntegrator=0  InitialConditionForFilter=0  DifferentiatorICPrevScaledInput=0  ExternalReset=none  TrackingMode=off  Kt=1  LimitOutput=off  SatLimitsSource=internal  UpperSaturationLimit=inf  LowerSaturationLimit=-inf  LinearizeAsGain=on  AntiWindupMode=none  Kb=1  LimitIntegrator=off  UpperIntegratorSaturationLimit=inf  LowerIntegratorSaturationLimit=-inf  POutMin=[]  POutMax=[]  IOutMin=[]  IOutMax=[]  DOutMin=[]  DOutMax=[]  NOutMin=[]  NOutMax=[]  SumOutMin=[]  SumOutMax=[]  SaturationOutMin=[]  SaturationOutMax=[]  PParamMin=[]  PParamMax=[]  IParamMin=[]  IParamMax=[]  DParamMin=[]  DParamMax=[]  NParamMin=[]  NParamMax=[]  KbParamMin=[]  KbParamMax=[]  KtParamMin=[]  KtParamMax=[]  KbOutMin=[]  KbOutMax=[]  KtOutMin=[]  KtOutMax=[]  IntegratorOutMin=[]  IntegratorOutMax=[]  FilterOutMin=[]  FilterOutMax=[]  SumI1OutMin=[]  SumI1OutMax=[]  SumI2OutMin=[]  SumI2OutMax=[]  SumI3OutMin=[]  SumI3OutMax=[]  SumI4OutMin=[]  SumI4OutMax=[]  SumDOutMin=[]  SumDOutMax=[]  DifferentiatorOutMin=[]  DifferentiatorOutMax=[]  FilterDiffOutCoefMin=[]  FilterDiffOutCoefMax=[]  ReciprocalOutMin=[]  ReciprocalOutMax=[]  SumDenOutMin=[]  SumDenOutMax=[]  SumNumOutMin=[]  SumNumOutMax=[]  DivideOutMin=[]  DivideOutMax=[]  UdiffTsProdOutMin=[]  UdiffTsProdOutMax=[]  NTsProdOutMin=[]  NTsProdOutMax=[]  UintegralTsProdOutMin=[]  UintegralTsProdOutMax=[]  UngainTsProdOutMin=[]  UngainTsProdOutMax=[]  ClampingZeroOutDataTypeStr=Inherit: Inherit via back propagation  ClampingZeroOutMin=[]  ClampingZeroOutMax=[]  FilterDenConstantOutDataTypeStr=Inherit: Inherit via back propagation  FilterDenConstantOutMin=[]  FilterDenConstantOutMax=[]  PCopyOutDataTypeStr=Inherit: Inherit via back propagation  PCopyOutMin=[]  PCopyOutMax=[]  NCopyOutDataTypeStr=Inherit: Inherit via back propagation  NCopyOutMin=[]  NCopyOutMax=[]  IntegratorContinuousStateAttributes=''  IntegratorStateMustResolveToSignalObject=off  IntegratorRTWStateStorageClass=Auto  FilterContinuousStateAttributes=''  FilterStateMustResolveToSignalObject=off  FilterRTWStateStorageClass=Auto  ParallelPVariant=InternalParameters  IdealPVariant=Disabled  IVariant=InternalParameters  DVariant=InternalParameters  IntegratorVariant=Continuous  SatVariant=Disabled  AWVariant=Passthrough  PCopyVariant=Disabled  TRVariant=Disabled  FdbkBlocksVariant=Forward  IdealPFdbkVariant=Disabled  SatFdbkVariant=Disabled  DerivativeFilterVariant=ContFilter  NVariant=InternalParameters  NCopyVariant=Disabled  FilterICVariant=InternalICsFilter  IntegratorICVariant=InternalICs  ExternalResetVariant=Disabled  TRSumVariant=Passthrough  SumFdbkVariant=Disabled  SumVariant=Sum_PID  TsampFilterVariant=InternalTs  TsampNgainVariant=Passthrough  TsampIntegralVariant=Disabled_SignalSpec  ExternalSaturationOutDataTypeStr=Inherit: Same as second input
  SVPWM Generator (2-Level) : spsSVPWMGenerator2LevelLib/SVPWM Generator (2-Level)  InputType=alpha-beta components  SwitchingPattern=Pattern #1  Fc=3000  ParUref=[0.8 -30 50]  Ts=0
  Scope : Scope  NumInputPorts=2
  Scope1 : Scope  NumInputPorts=2
  Scope2 : Scope  NumInputPorts=3
  Scope3 : Scope  NumInputPorts=2
  Sum : Sum  Inputs=|-+
  Sum1 : Sum  Inputs=|-+
  Terminator : Terminator
  Terminator1 : Terminator
  Terminator2 : Terminator
  WL1 : Gain  Gain=100*pi*(7e-3)
  WL2 : Gain  Gain=100*pi*(7e-3)
  abc to dq0 : spsabctodq0Lib/abc to dq0  Alignment=90 degrees behind phase A axis
  abc to dq1 : spsabctodq0Lib/abc to dq0  Alignment=90 degrees behind phase A axis
  dq0 to Alpha-Beta-Zero : spsdq0toAlphaBetaZeroLib/dq0 to Alpha-Beta-Zero  Alignment=90 degrees behind phase A axis
  iq* : Constant  Value=0
  SVPWM : Outport
  wires:
  SVPWM Generator (2-Level)/1 -> SVPWM/1
  Demux/1 -> Scope/1, SVPWM Generator (2-Level)/2
  Demux/2 -> Scope/2, SVPWM Generator (2-Level)/1
  Demux/3 -> Terminator/1
  dq0 to Alpha-Beta-Zero/1 -> Demux/1
  Mux/1 -> Gain/1
  Add/1 -> Scope2/1, Mux/1
  PID Controller/1 -> Scope2/3, Add/3
  Sum/1 -> PID Controller/1
  Demux1/3 -> Terminator1/1
  Demux1/1 -> Sum/1, Scope1/1, WL2/1
  Vabc/1 -> Scope3/1, abc to dq0/1
  Clock/1 -> Gain1/1
  Gain1/1 -> abc to dq1/2, dq0 to Alpha-Beta-Zero/2, abc to dq0/2
  Gain/1 -> dq0 to Alpha-Beta-Zero/1
  abc to dq1/1 -> Demux1/1
  Iabc/1 -> abc to dq1/1, Scope3/2
  Demux1/2 -> Scope1/2, WL1/1, Sum1/1
  iq*/1 -> Sum1/2
  Sum1/1 -> PID Controller1/1
  PID Controller1/1 -> Add1/3
  Add1/1 -> Mux/2
  0/1 -> Mux/3
  WL2/1 -> Add1/2
  id*/1 -> Sum/2
  WL1/1 -> Scope2/2, Add/2
  abc to dq0/1 -> Demux2/1
  Demux2/2 -> Add1/1
  Demux2/1 -> Add/1
  Demux2/3 -> Terminator2/1

== matlab function PMSG_Grid/MATLAB Function2 ==
  settings: updateMethod=DISCRETE
  data: t input; cst input; Vspeed output



%% 信号插值，连续

function Vspeed = Sink(t,cst)
    % 定义每个周期的持续时间
    T_array = [0.1, 0.15, 0.4, 0.05, 0.1, 0.2, 0.45, 0.1, 0.15, 0.3]; % 这十个周期的时间
    total_time = sum(T_array); % 确保总时间为2秒

    persistent amp_array;
    if isempty(amp_array)
        amp_array = [0.8, 0.2, 1, 0.5, 0.25, 0.6, 0.4, 0.3, 0.7, 0.15]; % 对应于10个周期的幅度
    end

    % 计算当前总周期数
    t_mod = mod(t, total_time); % 当前时间在总周期内的时间
    cumulative_time = 0;
    n = 0; % 当前周期编号

    % 找到当前时间属于哪个周期
    for i = 1:length(T_array)
        cumulative_time = cumulative_time + T_array(i);
        if t_mod < cumulative_time
            n = i;
            break;
        end
    end

    % 计算当前周期的相位
    if n == 1
        phase = t_mod / T_array(1);
    else
        phase = (t_mod - sum(T_array(1:n-1))) / T_array(n);
    end

    % 计算当前和下一个周期的幅度
    idx1 = mod(n - 1, length(amp_array)) + 1; % 当前周期幅度
    idx2 = mod(n, length(amp_array)) + 1; % 下一个周期幅度
    amp1 = amp_array(idx1);
    amp2 = amp_array(idx2);

    % 线性插值，保证信号连续
    amp = amp1 + (amp2 - amp1) * phase;
    Vspeed = cst + amp;
end



% function Vspeed = Sink(cst, t)
%     % 定义每个周期的持续时间
%     T_array = [0.2, 0.5, 0.3, 0.15, 0.55]; % 这五个周期的时间
%     total_time = sum(T_array); % 确保总时间为2秒
% 
%     persistent amp_array;
%     if isempty(amp_array)
%         amp_array = [0.8, 0.2, 1, 0.5, 0.25];
%     end
% 
%     % 计算当前总周期数
%     t_mod = mod(t, total_time); % 当前时间在总周期内的时间
%     cumulative_time = 0;
%     n = 0; % 当前周期编号
% 
%     % 找到当前时间属于哪个周期
%     for i = 1:length(T_array)
%         cumulative_time = cumulative_time + T_array(i);
%         if t_mod < cumulative_time
%             n = i;
%             break;
%         end
%     end
% 
%     % 计算当前周期的相位
%     if n == 1
%         phase = t_mod / T_array(1);
%     else
%         phase = (t_mod - sum(T_array(1:n-1))) / T_array(n);
%     end
% 
%     % 计算当前和下一个周期的幅度
%     idx1 = mod(n - 1, length(amp_array)) + 1; % 当前周期幅度
%     idx2 = mod(n, length(amp_array)) + 1; % 下一个周期幅度
%     amp1 = amp_array(idx1);
%     amp2 = amp_array(idx2);
% 
%     % 线性插值，保证信号连续
%     amp = amp1 + (amp2 - amp1) * phase;
%     Vspeed = cst + amp;
% end
